simulink model "basic_serial_send_Uint8"  (R2018a)
settings: Solver=ode4  StartTime=0.0  StopTime=10.0  FixedStep=1  RelTol=1e-3
undefined symbols (not defined in the file or in its folder): LF, serial
libraries: instrumentlib x2
settings Model: EnablePacing=on  Creator=shiib  LastModifiedBy=takada

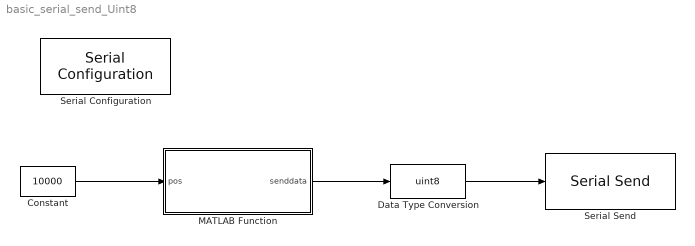
== system basic_serial_send_Uint8 ==
  Constant : Constant  Value=10000  OutDataTypeStr=uint16  SampleTime=1
  Data Type Conversion : DataTypeConversion  OutDataTypeStr=uint8
  MATLAB Function : MATLAB Function  TreatAsAtomicUnit=on
  Serial Configuration : instrumentlib/Serial Configuration  Priority=-200000  ComPortMenu=COM1  ComPort=COM1  ObjConstructor=serial('COM1');  BaudRate=115200  DataBits=8  Parity=none  StopBits=1  FlowControl=none  Timeout=10  ByteOrder=LittleEndian
  Serial Send : instrumentlib/Serial Send  ComPortMenu=COM1  ComPort=COM1  ObjConstructor=serial('COM1');  Terminator=LF ('\n')  EnableBlockingMode=on
  wires:
  Constant/1 -> MATLAB Function/1(pos)
  MATLAB Function/1(senddata) -> Data Type Conversion/1
  Data Type Conversion/1 -> Serial Send/1

== matlab function basic_serial_send_Uint8/MATLAB Function ==
  data: pos input; senddata output
% script_sendTargetPosition
% MATLAB EPOS LibraryのsendTargetPosition()から書き換え

% function [] = sendTargetPosition( obj, pos )

function senddata = func_sendTargetPosition(pos)
% pos = 20480;

%Sets the TargetPosition for Profile Position mode
%pos must be an integer.
pos_hex = '';

if pos >= 0
    pos_hex = dec2hex(pos, 8);
else
    pos_hex = dec2hex(2^32+pos, 8);
end

%% Build write object request frame EPOS Node 1
%opCode(write): 0x11
%Len-1: 3
%object index(Target Position): 0x607A
%subindex and nodeID: 0x0100
%BYTE Data[4]: pos_hex(1:4), pos_hex(5:8)


%opCode = uint16(myhex2dec('11'));
opCode = uint16(17);
Len_1 = uint16(3);
%DATA = uint16([myhex2dec('7A') myhex2dec('60') myhex2dec('00') myhex2dec('01') myhex2dec(pos_hex(7:8)) myhex2dec(pos_hex(5:6)) myhex2dec(pos_hex(3:4)) myhex2dec(pos_hex(1:2)) ]);
DATA = uint16([122 96 0 1 myhex2dec(pos_hex(7:8)) myhex2dec(pos_hex(5:6)) myhex2dec(pos_hex(3:4)) myhex2dec(pos_hex(1:2)) ]);
%DATAforCRC = uint16([myhex2dec('1103') myhex2dec('607A') myhex2dec('0100') myhex2dec(pos_hex(5:8)) myhex2dec(pos_hex(1:4)) myhex2dec('0000')]);
DATAforCRC = uint16([4355 24698 256 myhex2dec(pos_hex(5:8)) myhex2dec(pos_hex(1:4)) 0]);
numberofWordsCRC = 6;
crc_hex = dec2hex(CRCcalc(DATAforCRC, numberofWordsCRC),4);
CRC = uint16([myhex2dec(crc_hex(3:4)) myhex2dec(crc_hex(1:2))]);

% fwrite(obj,opCode); %Send the opCode
% ReadyAck = fread(obj, 1); %See if EPOS is ready
% if ReadyAck == 'O'
%     %Now send the data
%     fwrite(obj,[Len_1 DATA CRC]); 
%    
%     EndAck = fread(obj, 1); %See if EPOS is ready
%     if EndAck ~= 'O'
%        warning('EPOS did not send correct EndAck');
%     end
% 
%     fwrite(obj,char('O'));%tell epos to send his response (error code)
%     
%     
%     
%     out = fread(obj, 8); %read from input buffer
%     
%     if CRCcheck(out)
%         fwrite(obj,char('O'));
%         disp('Checksum good')
%     else
%         warning('Bad Checksum')
%     end
%     
% elseif ReadyAck == 'F'
%     disp('EPOS ReadyAck = F')
% else
%     error('Error at reading ReadyAck')
% end

% fwrite(obj, [opCode Len_1 DATA CRC char('O')]) %send all at once
% senddata=[opCode Len_1 DATA CRC 79];
% senddata=[opCode Len_1 DATA CRC char('O')];
senddata=[opCode Len_1 DATA CRC];
% 16進数でsprintf
% sprintf('%x',senddata)

% 以下はとりあえず削除
